simulink model "IEEE9_case"  (R2024b)
settings: Solver=FixedStepAuto  StartTime=0  StopTime=5  FixedStep=1e-7  RelTol=1e-3
values from neighbouring files (symbols this model uses):
  SG_D_1_D = 0.01056    [IEEE9_case_parameters.m]    (also in case1_parameters.m; case2_parameters.m; case3_parameters.m; case4_parameters.m)
  SG_D_1_EnableSaturation = 0    [IEEE9_case_parameters.m]    (also in case1_parameters.m; case2_parameters.m; case3_parameters.m; case4_parameters.m)
  SG_D_1_f0 = 60    [IEEE9_case_parameters.m]    (also in case1_parameters.m; case2_parameters.m; case3_parameters.m; case4_parameters.m)
  SG_D_1_H = 7.5    [IEEE9_case_parameters.m]    (also in case1_parameters.m; case2_parameters.m; case3_parameters.m; case4_parameters.m)
  SG_D_1_K_A = 20    [IEEE9_case_parameters.m]    (also in case1_parameters.m; case2_parameters.m; case3_parameters.m; case4_parameters.m)
  SG_D_1_K_E = 1.000000e+1    (= 10)    [IEEE9_case_parameters.m]    (also in case1_parameters.m; case2_parameters.m; case3_parameters.m; case4_parameters.m)
  SG_D_1_K_F = 2.363    [IEEE9_case_parameters.m]    (also in case1_parameters.m; case2_parameters.m; case3_parameters.m; case4_parameters.m)
  SG_D_1_K_s = 0.5    [IEEE9_case_parameters.m]    (also in case1_parameters.m = 5; case2_parameters.m = 5; case3_parameters.m = 5; case4_parameters.m = 5)
  SG_D_1_R_a = 0.001088    [IEEE9_case_parameters.m]    (also in case1_parameters.m; case2_parameters.m; case3_parameters.m; case4_parameters.m)
  SG_D_1_S_A = 1    [IEEE9_case_parameters.m]    (also in case1_parameters.m; case2_parameters.m; case3_parameters.m; case4_parameters.m)
  SG_D_1_S_B = 0.103    [IEEE9_case_parameters.m]    (also in case1_parameters.m; case2_parameters.m; case3_parameters.m; case4_parameters.m)
  SG_D_1_S_N = 10.659857    [IEEE9_case_parameters.m]    (also in case1_parameters.m; case2_parameters.m; case3_parameters.m; case4_parameters.m)
  SG_D_1_SpeedPara = 200    [IEEE9_case_parameters.m]    (also in case1_parameters.m; case2_parameters.m; case3_parameters.m; case4_parameters.m)
  SG_D_1_T_0 = 0.720173    [IEEE9_case_parameters.m]    (also in case1_parameters.m = 0.755522; case2_parameters.m = 0.808931; case3_parameters.m = 0.869402; case4_parameters.m = 0.729316)
  SG_D_1_T_1 = 0.3    [IEEE9_case_parameters.m]    (also in case1_parameters.m; case2_parameters.m; case3_parameters.m; case4_parameters.m)
  SG_D_1_T_2 = 0.05    [IEEE9_case_parameters.m]    (also in case1_parameters.m; case2_parameters.m; case3_parameters.m; case4_parameters.m)
  SG_D_1_T_3 = 0.02    [IEEE9_case_parameters.m]    (also in case1_parameters.m; case2_parameters.m; case3_parameters.m; case4_parameters.m)
  SG_D_1_T_4 = 0.005    [IEEE9_case_parameters.m]    (also in case1_parameters.m; case2_parameters.m; case3_parameters.m; case4_parameters.m)
  SG_D_1_T_A = 0.02    [IEEE9_case_parameters.m]    (also in case1_parameters.m; case2_parameters.m; case3_parameters.m; case4_parameters.m)
  SG_D_1_T_dd = 8.000000e+0    (= 8)    [IEEE9_case_parameters.m]    (also in case1_parameters.m; case2_parameters.m; case3_parameters.m; case4_parameters.m)
  SG_D_1_T_ddd = 0.04    [IEEE9_case_parameters.m]    (also in case1_parameters.m; case2_parameters.m; case3_parameters.m; case4_parameters.m)
  SG_D_1_T_E = 0.314    [IEEE9_case_parameters.m]    (also in case1_parameters.m; case2_parameters.m; case3_parameters.m; case4_parameters.m)
  SG_D_1_T_F = 0.35    [IEEE9_case_parameters.m]    (also in case1_parameters.m; case2_parameters.m; case3_parameters.m; case4_parameters.m)
  SG_D_1_T_qd = 0.8    [IEEE9_case_parameters.m]    (also in case1_parameters.m; case2_parameters.m; case3_parameters.m; case4_parameters.m)
  SG_D_1_T_qdd = 0.02    [IEEE9_case_parameters.m]    (also in case1_parameters.m; case2_parameters.m; case3_parameters.m; case4_parameters.m)
  SG_D_1_T_speed = 0.1    [IEEE9_case_parameters.m]    (also in case1_parameters.m = 200; case2_parameters.m = 200; case3_parameters.m = 200; case4_parameters.m = 200)
  SG_D_1_T_w = 0.5    [IEEE9_case_parameters.m]    (also in case1_parameters.m; case2_parameters.m; case3_parameters.m; case4_parameters.m)
  SG_D_1_V_ref = 1.990276    [IEEE9_case_parameters.m]    (also in case1_parameters.m = 2.042296; case2_parameters.m = 2.051388; case3_parameters.m = 2.089584; case4_parameters.m = 2.01845)
  SG_D_1_w_ref = 376.991118    [IEEE9_case_parameters.m]    (also in case1_parameters.m; case2_parameters.m; case3_parameters.m; case4_parameters.m)
  SG_D_1_wb = 6.000000e+1    (= 60)    [IEEE9_case_parameters.m]    (also in case1_parameters.m; case2_parameters.m; case3_parameters.m; case4_parameters.m)
  SG_D_1_x_d = 1.9    [IEEE9_case_parameters.m]    (also in case1_parameters.m; case2_parameters.m; case3_parameters.m; case4_parameters.m)
  SG_D_1_x_dd = 0.302    [IEEE9_case_parameters.m]    (also in case1_parameters.m; case2_parameters.m; case3_parameters.m; case4_parameters.m)
  SG_D_1_x_ddd = 0.204    [IEEE9_case_parameters.m]    (also in case1_parameters.m; case2_parameters.m; case3_parameters.m; case4_parameters.m)
  SG_D_1_x_l = 0.05    [IEEE9_case_parameters.m]    (also in case1_parameters.m; case2_parameters.m; case3_parameters.m; case4_parameters.m)
  SG_D_1_x_q = 1.3    [IEEE9_case_parameters.m]    (also in case1_parameters.m; case2_parameters.m; case3_parameters.m; case4_parameters.m)
  SG_D_1_x_qd = 0.5    [IEEE9_case_parameters.m]    (also in case1_parameters.m; case2_parameters.m; case3_parameters.m; case4_parameters.m)
  SG_D_1_x_qdd = 0.3    [IEEE9_case_parameters.m]    (also in case1_parameters.m; case2_parameters.m; case3_parameters.m; case4_parameters.m)
  SG_D_2_D = 0.02    [IEEE9_case_parameters.m]    (also in case1_parameters.m; case2_parameters.m; case3_parameters.m; case4_parameters.m)
  SG_D_2_EnableSaturation = 0    [IEEE9_case_parameters.m]    (also in case1_parameters.m; case2_parameters.m; case3_parameters.m; case4_parameters.m)
  SG_D_2_f0 = 60    [IEEE9_case_parameters.m]    (also in case1_parameters.m; case2_parameters.m; case3_parameters.m; case4_parameters.m)
  SG_D_2_H = 8.000000e+0    (= 8)    [IEEE9_case_parameters.m]    (also in case1_parameters.m; case2_parameters.m; case3_parameters.m; case4_parameters.m)
  SG_D_2_K_A = 20    [IEEE9_case_parameters.m]    (also in case1_parameters.m; case2_parameters.m; case3_parameters.m; case4_parameters.m)
  SG_D_2_K_E = 1.000000e+1    (= 10)    [IEEE9_case_parameters.m]    (also in case1_parameters.m; case2_parameters.m; case3_parameters.m; case4_parameters.m)
  SG_D_2_K_F = 2.363    [IEEE9_case_parameters.m]    (also in case1_parameters.m; case2_parameters.m; case3_parameters.m; case4_parameters.m)
  SG_D_2_K_s = 0.5    [IEEE9_case_parameters.m]    (also in case1_parameters.m = 4; case2_parameters.m = 4; case3_parameters.m = 4; case4_parameters.m = 4)
  SG_D_2_R_a = 0.001088    [IEEE9_case_parameters.m]    (also in case1_parameters.m; case2_parameters.m; case3_parameters.m; case4_parameters.m)
  SG_D_2_S_A = 1    [IEEE9_case_parameters.m]    (also in case1_parameters.m; case2_parameters.m; case3_parameters.m; case4_parameters.m)
  SG_D_2_S_B = 0.103    [IEEE9_case_parameters.m]    (also in case1_parameters.m; case2_parameters.m; case3_parameters.m; case4_parameters.m)
  SG_D_2_S_N = 10.659857    [IEEE9_case_parameters.m]    (also in case1_parameters.m; case2_parameters.m; case3_parameters.m; case4_parameters.m)
  SG_D_2_SpeedPara = 200    [IEEE9_case_parameters.m]    (also in case1_parameters.m; case2_parameters.m; case3_parameters.m; case4_parameters.m)
  SG_D_2_T_0 = 1.632913    [IEEE9_case_parameters.m]    (also in case1_parameters.m = 1.632925; case2_parameters.m = 1.632915; case3_parameters.m = 1.632914; case4_parameters.m = 1.632927)
  SG_D_2_T_1 = 0.2    [IEEE9_case_parameters.m]    (also in case1_parameters.m; case2_parameters.m; case3_parameters.m; case4_parameters.m)
  SG_D_2_T_2 = 0.05    [IEEE9_case_parameters.m]    (also in case1_parameters.m; case2_parameters.m; case3_parameters.m; case4_parameters.m)
  SG_D_2_T_3 = 0.02    [IEEE9_case_parameters.m]    (also in case1_parameters.m; case2_parameters.m; case3_parameters.m; case4_parameters.m)
  SG_D_2_T_4 = 0.005    [IEEE9_case_parameters.m]    (also in case1_parameters.m; case2_parameters.m; case3_parameters.m; case4_parameters.m)
  SG_D_2_T_A = 0.02    [IEEE9_case_parameters.m]    (also in case1_parameters.m; case2_parameters.m; case3_parameters.m; case4_parameters.m)
  SG_D_2_T_dd = 7.9    [IEEE9_case_parameters.m]    (also in case1_parameters.m; case2_parameters.m; case3_parameters.m; case4_parameters.m)
  SG_D_2_T_ddd = 0.04    [IEEE9_case_parameters.m]    (also in case1_parameters.m; case2_parameters.m; case3_parameters.m; case4_parameters.m)
  SG_D_2_T_E = 0.314    [IEEE9_case_parameters.m]    (also in case1_parameters.m; case2_parameters.m; case3_parameters.m; case4_parameters.m)
  SG_D_2_T_F = 0.35    [IEEE9_case_parameters.m]    (also in case1_parameters.m; case2_parameters.m; case3_parameters.m; case4_parameters.m)
  SG_D_2_T_qd = 0.8    [IEEE9_case_parameters.m]    (also in case1_parameters.m; case2_parameters.m; case3_parameters.m; case4_parameters.m)
  SG_D_2_T_qdd = 0.015    [IEEE9_case_parameters.m]    (also in case1_parameters.m; case2_parameters.m; case3_parameters.m; case4_parameters.m)
  SG_D_2_T_speed = 0.1    [IEEE9_case_parameters.m]    (also in case1_parameters.m = 150; case2_parameters.m = 150; case3_parameters.m = 150; case4_parameters.m = 150)
  SG_D_2_T_w = 0.35    [IEEE9_case_parameters.m]    (also in case1_parameters.m; case2_parameters.m; case3_parameters.m; case4_parameters.m)
  SG_D_2_V_ref = 2.58547    [IEEE9_case_parameters.m]    (also in case1_parameters.m = 2.597896; case2_parameters.m = 2.587136; case3_parameters.m = 2.586042; case4_parameters.m = 2.599679)
  SG_D_2_w_ref = 376.991118    [IEEE9_case_parameters.m]    (also in case1_parameters.m; case2_parameters.m; case3_parameters.m; case4_parameters.m)
  SG_D_2_wb = 6.000000e+1    (= 60)    [IEEE9_case_parameters.m]    (also in case1_parameters.m; case2_parameters.m; case3_parameters.m; case4_parameters.m)
  SG_D_2_x_d = 1.8    [IEEE9_case_parameters.m]    (also in case1_parameters.m; case2_parameters.m; case3_parameters.m; case4_parameters.m)
  SG_D_2_x_dd = 0.302    [IEEE9_case_parameters.m]    (also in case1_parameters.m; case2_parameters.m; case3_parameters.m; case4_parameters.m)
  SG_D_2_x_ddd = 0.204    [IEEE9_case_parameters.m]    (also in case1_parameters.m; case2_parameters.m; case3_parameters.m; case4_parameters.m)
  SG_D_2_x_l = 0.05    [IEEE9_case_parameters.m]    (also in case1_parameters.m; case2_parameters.m; case3_parameters.m; case4_parameters.m)
  SG_D_2_x_q = 1.25    [IEEE9_case_parameters.m]    (also in case1_parameters.m; case2_parameters.m; case3_parameters.m; case4_parameters.m)
  SG_D_2_x_qd = 0.5    [IEEE9_case_parameters.m]    (also in case1_parameters.m; case2_parameters.m; case3_parameters.m; case4_parameters.m)
  SG_D_2_x_qdd = 0.3    [IEEE9_case_parameters.m]    (also in case1_parameters.m; case2_parameters.m; case3_parameters.m; case4_parameters.m)
  SG_D_3_D = 0.02    [IEEE9_case_parameters.m]    (also in case1_parameters.m; case2_parameters.m; case3_parameters.m; case4_parameters.m)
  SG_D_3_EnableSaturation = 0    [IEEE9_case_parameters.m]    (also in case1_parameters.m; case2_parameters.m; case3_parameters.m; case4_parameters.m)
  SG_D_3_f0 = 60    [IEEE9_case_parameters.m]    (also in case1_parameters.m; case2_parameters.m; case3_parameters.m; case4_parameters.m)
  SG_D_3_H = 7.7    [IEEE9_case_parameters.m]    (also in case1_parameters.m; case2_parameters.m; case3_parameters.m; case4_parameters.m)
  SG_D_3_K_A = 20    [IEEE9_case_parameters.m]    (also in case1_parameters.m; case2_parameters.m; case3_parameters.m; case4_parameters.m)
  SG_D_3_K_E = 1.000000e+1    (= 10)    [IEEE9_case_parameters.m]    (also in case1_parameters.m; case2_parameters.m; case3_parameters.m; case4_parameters.m)
  SG_D_3_K_F = 2.363    [IEEE9_case_parameters.m]    (also in case1_parameters.m; case2_parameters.m; case3_parameters.m; case4_parameters.m)
  SG_D_3_K_s = 0.2    [IEEE9_case_parameters.m]    (also in case1_parameters.m = 2; case2_parameters.m = 2; case3_parameters.m = 2; case4_parameters.m = 2)
  SG_D_3_R_a = 0.001088    [IEEE9_case_parameters.m]    (also in case1_parameters.m; case2_parameters.m; case3_parameters.m; case4_parameters.m)
  SG_D_3_S_A = 1    [IEEE9_case_parameters.m]    (also in case1_parameters.m; case2_parameters.m; case3_parameters.m; case4_parameters.m)
  SG_D_3_S_B = 0.103    [IEEE9_case_parameters.m]    (also in case1_parameters.m; case2_parameters.m; case3_parameters.m; case4_parameters.m)
  SG_D_3_S_N = 10.659857    [IEEE9_case_parameters.m]    (also in case1_parameters.m; case2_parameters.m; case3_parameters.m; case4_parameters.m)
  SG_D_3_SpeedPara = 200    [IEEE9_case_parameters.m]    (also in case1_parameters.m; case2_parameters.m; case3_parameters.m; case4_parameters.m)
  SG_D_3_T_0 = 0.850788    [IEEE9_case_parameters.m]    (also in case1_parameters.m = 0.850786; case2_parameters.m = 0.850787; case3_parameters.m; case4_parameters.m = 0.850786)
  SG_D_3_T_1 = 0.2    [IEEE9_case_parameters.m]    (also in case1_parameters.m; case2_parameters.m; case3_parameters.m; case4_parameters.m)
  SG_D_3_T_2 = 0.05    [IEEE9_case_parameters.m]    (also in case1_parameters.m; case2_parameters.m; case3_parameters.m; case4_parameters.m)
  SG_D_3_T_3 = 0.02    [IEEE9_case_parameters.m]    (also in case1_parameters.m; case2_parameters.m; case3_parameters.m; case4_parameters.m)
  SG_D_3_T_4 = 0.005    [IEEE9_case_parameters.m]    (also in case1_parameters.m; case2_parameters.m; case3_parameters.m; case4_parameters.m)
  SG_D_3_T_A = 0.02    [IEEE9_case_parameters.m]    (also in case1_parameters.m; case2_parameters.m; case3_parameters.m; case4_parameters.m)
  SG_D_3_T_dd = 8.1    [IEEE9_case_parameters.m]    (also in case1_parameters.m; case2_parameters.m; case3_parameters.m; case4_parameters.m)
  SG_D_3_T_ddd = 0.04    [IEEE9_case_parameters.m]    (also in case1_parameters.m; case2_parameters.m; case3_parameters.m; case4_parameters.m)
  SG_D_3_T_E = 0.314    [IEEE9_case_parameters.m]    (also in case1_parameters.m; case2_parameters.m; case3_parameters.m; case4_parameters.m)
  SG_D_3_T_F = 0.35    [IEEE9_case_parameters.m]    (also in case1_parameters.m; case2_parameters.m; case3_parameters.m; case4_parameters.m)
  SG_D_3_T_qd = 0.8    [IEEE9_case_parameters.m]    (also in case1_parameters.m; case2_parameters.m; case3_parameters.m; case4_parameters.m)
  SG_D_3_T_qdd = 0.015    [IEEE9_case_parameters.m]    (also in case1_parameters.m; case2_parameters.m; case3_parameters.m; case4_parameters.m)
  SG_D_3_T_speed = 0.1    [IEEE9_case_parameters.m]    (also in case1_parameters.m = 180; case2_parameters.m = 180; case3_parameters.m = 180; case4_parameters.m = 180)
  SG_D_3_T_w = 0.4    [IEEE9_case_parameters.m]    (also in case1_parameters.m; case2_parameters.m; case3_parameters.m; case4_parameters.m)
  SG_D_3_V_ref = 1.892727    [IEEE9_case_parameters.m]    (also in case1_parameters.m = 1.906439; case2_parameters.m = 1.895535; case3_parameters.m = 1.892105; case4_parameters.m = 1.906598)
  SG_D_3_w_ref = 376.991118    [IEEE9_case_parameters.m]    (also in case1_parameters.m; case2_parameters.m; case3_parameters.m; case4_parameters.m)
  SG_D_3_wb = 6.000000e+1    (= 60)    [IEEE9_case_parameters.m]    (also in case1_parameters.m; case2_parameters.m; case3_parameters.m; case4_parameters.m)
  SG_D_3_x_d = 1.85    [IEEE9_case_parameters.m]    (also in case1_parameters.m; case2_parameters.m; case3_parameters.m; case4_parameters.m)
  SG_D_3_x_dd = 0.302    [IEEE9_case_parameters.m]    (also in case1_parameters.m; case2_parameters.m; case3_parameters.m; case4_parameters.m)
  SG_D_3_x_ddd = 0.204    [IEEE9_case_parameters.m]    (also in case1_parameters.m; case2_parameters.m; case3_parameters.m; case4_parameters.m)
  SG_D_3_x_l = 0.05    [IEEE9_case_parameters.m]    (also in case1_parameters.m; case2_parameters.m; case3_parameters.m; case4_parameters.m)
  SG_D_3_x_q = 1.2    [IEEE9_case_parameters.m]    (also in case1_parameters.m; case2_parameters.m; case3_parameters.m; case4_parameters.m)
  SG_D_3_x_qd = 0.5    [IEEE9_case_parameters.m]    (also in case1_parameters.m; case2_parameters.m; case3_parameters.m; case4_parameters.m)
  SG_D_3_x_qdd = 0.3    [IEEE9_case_parameters.m]    (also in case1_parameters.m; case2_parameters.m; case3_parameters.m; case4_parameters.m)
(part 11 of 12)

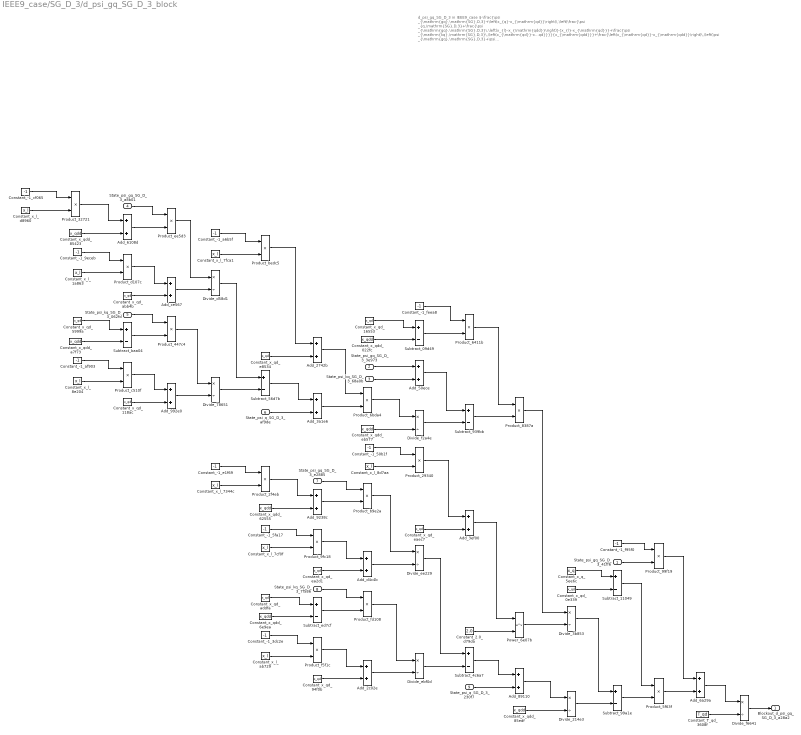
== system IEEE9_case/SG_D_3/d_psi_gq_SG_D_3_block ==
  note: d_psi_gq_SG_D_3 in IEEE9_case
      | $-\frac{\psi _{\mathrm{gq},\mathrm{SG},D,3}+\left(x_{q}-x_{\mathrm{qd}}\right)\,\left(\frac{\psi _{q,\mathrm{SG},D,3}+\frac{\psi _{\mathrm{gq},\mathrm{SG},D,3}\,\left(x_{l}-x_{\mathrm{qdd}}\right)}{x_{l}-x_{\mathrm{qd}}}+\frac{\psi _{\mathrm{kq},\mathrm{SG},D,3}\,\left(x_{\mathrm{qd}}-x_{\mathrm{qdd}}\right)}{x_{l}-x_{\mathrm{qd}}}}{x_{\mathrm{qdd}}}+\frac{\left(x_{\mathrm{qd}}-x_{\mathrm{qdd}}\right)\,\left(\psi _{\mathrm{gq},\mathrm{SG},D,3}+\psi _{\mathrm{kq},\mathrm{SG},D,3}+\frac{\left(x_{l}-x_{\mathrm{qd}}\right)\,\left(\psi _{q,\mathrm{SG},D,3}+\frac{\psi _{\mathrm{gq},\mathrm{SG},D,3}\,\left(x_{l}-x_{\mathrm{qdd}}\right)}{x_{l}-x_{\mathrm{qd}}}+\frac{\psi _{\mathrm{kq},\mathrm{SG},D,3}\,\left(x_{\mathrm{qd}}-x_{\mathrm{qdd}}\right)}{x_{l}-x_{\mathrm{qd}}}\right)}{x_{\mathrm{qdd}}}\right)}{{\left(x_{l}-x_{\mathrm{qd}}\right)}^2}\right)}{T_{\mathrm{qd}}}$
      | Automatically generated on 2025-11-01 08:49:54 .
  State_psi_gq_SG_D_3_41ff6 : Inport
  State_psi_gq_SG_D_3_3e973 : Inport  Port=2
  State_psi_kq_SG_D_3_68a0b : Inport  Port=3
  State_psi_gq_SG_D_3_a8b01 : Inport  Port=4
  State_psi_kq_SG_D_3_062fd : Inport  Port=5
  State_psi_q_SG_D_3_af9de : Inport  Port=6
  State_psi_gq_SG_D_3_e2885 : Inport  Port=7
  State_psi_kq_SG_D_3_7f586 : Inport  Port=8
  State_psi_q_SG_D_3_230f7 : Inport  Port=9
  Add_2742b : Sum
  Add_2c02e : Sum
  Add_3a1e6 : Sum
  Add_3ef00 : Sum
  Add_50ece : Sum
  Add_6108d : Sum
  Add_6a29a : Sum
  Add_89110 : Sum
  Add_9238c : Sum
  Add_992e0 : Sum
  Add_ce567 : Sum
  Add_d4c4b : Sum
  Constant_-1_3dc2e : Constant  Value=-1
  Constant_-1_50b1f : Constant  Value=-1
  Constant_-1_5fa17 : Constant  Value=-1
  Constant_-1_9eceb : Constant  Value=-1
  Constant_-1_a6b5f : Constant  Value=-1
  Constant_-1_af903 : Constant  Value=-1
  Constant_-1_cf065 : Constant  Value=-1
  Constant_-1_e1f69 : Constant  Value=-1
  Constant_-1_f95f0 : Constant  Value=-1
  Constant_-1_feea8 : Constant  Value=-1
  Constant_2.0_d79da : Constant  Value=2.0
  Constant_T_qd_3608f : Constant  Value=T_qd
  Constant_x_l_1a863 : Constant  Value=x_l
  Constant_x_l_7344c : Constant  Value=x_l
  Constant_x_l_7cf0f : Constant  Value=x_l
  Constant_x_l_7fca1 : Constant  Value=x_l
  Constant_x_l_8d7aa : Constant  Value=x_l
  Constant_x_l_8e204 : Constant  Value=x_l
  Constant_x_l_ab729 : Constant  Value=x_l
  Constant_x_l_d8960 : Constant  Value=x_l
  Constant_x_q_5ee6c : Constant  Value=x_q
  Constant_x_qd_0e339 : Constant  Value=x_qd
  Constant_x_qd_118ac : Constant  Value=x_qd
  Constant_x_qd_16553 : Constant  Value=x_qd
  Constant_x_qd_5999a : Constant  Value=x_qd
  Constant_x_qd_94f0b : Constant  Value=x_qd
  Constant_x_qd_abb4b : Constant  Value=x_qd
  Constant_x_qd_addfa : Constant  Value=x_qd
  Constant_x_qd_e8534 : Constant  Value=x_qd
  Constant_x_qd_ea2d1 : Constant  Value=x_qd
  Constant_x_qd_eaec7 : Constant  Value=x_qd
  Constant_x_qdd_022fc : Constant  Value=x_qdd
  Constant_x_qdd_62555 : Constant  Value=x_qdd
  Constant_x_qdd_6e9ea : Constant  Value=x_qdd
  Constant_x_qdd_85423 : Constant  Value=x_qdd
  Constant_x_qdd_85edf : Constant  Value=x_qdd
  Constant_x_qdd_a7f73 : Constant  Value=x_qdd
  Constant_x_qdd_eb577 : Constant  Value=x_qdd
  Divide_214e3 : Product  Inputs=*/
  Divide_3b853 : Product  Inputs=*/
  Divide_78651 : Product  Inputs=*/
  Divide_d58d1 : Product  Inputs=*/
  Divide_ebf0d : Product  Inputs=*/
  Divide_ee229 : Product  Inputs=*/
  Divide_f2a4e : Product  Inputs=*/
  Divide_f6641 : Product  Inputs=*/
  Power_6e07b : Math  Operator=pow
  Product_29340 : Product
  Product_2f4eb : Product
  Product_32721 : Product
  Product_447c4 : Product
  Product_5f63f : Product
  Product_6411b : Product
  Product_6bda4 : Product
  Product_8387a : Product
  Product_99f19 : Product
  Product_9fc18 : Product
  Product_b9e2a : Product
  Product_bedc5 : Product
  Product_c510f : Product
  Product_d107c : Product
  Product_ee5d3 : Product
  Product_f5f1c : Product
  Product_fd108 : Product
  Subtract_09d49 : Sum  Inputs=+-
  Subtract_11049 : Sum  Inputs=+-
  Subtract_4c6a7 : Sum  Inputs=+-
  Subtract_56d7b : Sum  Inputs=+-
  Subtract_939bb : Sum  Inputs=+-
  Subtract_99a1e : Sum  Inputs=+-
  Subtract_baa04 : Sum  Inputs=+-
  Subtract_ed7cf : Sum  Inputs=+-
  Blockout_d_psi_gq_SG_D_3_a28a2 : Outport
  wires:
  Constant_x_l_8d7aa/1 -> Product_29340/2
  Constant_x_qd_5999a/1 -> Subtract_baa04/1
  Add_2742b/1 -> Product_6bda4/1
  Constant_-1_cf065/1 -> Product_32721/1
  Add_6108d/1 -> Product_ee5d3/2
  Constant_x_qdd_a7f73/1 -> Subtract_baa04/2
  Constant_x_qd_e8534/1 -> Add_2742b/2
  Constant_x_l_d8960/1 -> Product_32721/2
  Constant_x_l_1a863/1 -> Product_d107c/2
  Add_2c02e/1 -> Divide_ebf0d/2
  State_psi_kq_SG_D_3_68a0b/1 -> Add_50ece/2
  Constant_x_qdd_85423/1 -> Add_6108d/2
  Product_32721/1 -> Add_6108d/1
  Constant_x_qd_94f0b/1 -> Add_2c02e/2
  Product_6411b/1 -> Product_8387a/1
  Constant_-1_e1f69/1 -> Product_2f4eb/1
  Constant_-1_9eceb/1 -> Product_d107c/1
  Constant_-1_af903/1 -> Product_c510f/1
  Constant_x_l_8e204/1 -> Product_c510f/2
  Constant_-1_feea8/1 -> Product_6411b/1
  Constant_-1_f95f0/1 -> Product_99f19/1
  State_psi_gq_SG_D_3_a8b01/1 -> Product_ee5d3/1
  Product_2f4eb/1 -> Add_9238c/1
  Product_d107c/1 -> Add_ce567/1
  Product_f5f1c/1 -> Add_2c02e/1
  Constant_x_qd_abb4b/1 -> Add_ce567/2
  Constant_-1_5fa17/1 -> Product_9fc18/1
  State_psi_kq_SG_D_3_062fd/1 -> Product_447c4/1
  Subtract_baa04/1 -> Product_447c4/2
  Product_c510f/1 -> Add_992e0/1
  Add_9238c/1 -> Product_b9e2a/2
  Add_ce567/1 -> Divide_d58d1/2
  Constant_x_qd_118ac/1 -> Add_992e0/2
  Product_ee5d3/1 -> Divide_d58d1/1
  Constant_T_qd_3608f/1 -> Divide_f6641/2
  Product_9fc18/1 -> Add_d4c4b/1
  Product_447c4/1 -> Divide_78651/1
  Product_fd108/1 -> Divide_ebf0d/1
  Add_992e0/1 -> Divide_78651/2
  Constant_-1_a6b5f/1 -> Product_bedc5/1
  Constant_x_qdd_eb577/1 -> Divide_f2a4e/2
  Constant_x_l_7fca1/1 -> Product_bedc5/2
  Divide_d58d1/1 -> Subtract_56d7b/1
  Constant_x_qd_0e339/1 -> Subtract_11049/2
  Add_d4c4b/1 -> Divide_ee229/2
  Divide_78651/1 -> Subtract_56d7b/2
  Constant_x_l_7344c/1 -> Product_2f4eb/2
  Product_bedc5/1 -> Add_2742b/1
  Constant_-1_50b1f/1 -> Product_29340/1
  Constant_x_l_7cf0f/1 -> Product_9fc18/2
  Subtract_56d7b/1 -> Add_3a1e6/1
  State_psi_q_SG_D_3_af9de/1 -> Add_3a1e6/2
  Constant_-1_3dc2e/1 -> Product_f5f1c/1
  Constant_x_qdd_62555/1 -> Add_9238c/2
  Constant_x_qd_addfa/1 -> Subtract_ed7cf/1
  Constant_x_qdd_6e9ea/1 -> Subtract_ed7cf/2
  Constant_x_l_ab729/1 -> Product_f5f1c/2
  Add_3a1e6/1 -> Product_6bda4/2
  Constant_x_qdd_022fc/1 -> Subtract_09d49/2
  State_psi_gq_SG_D_3_e2885/1 -> Product_b9e2a/1
  Constant_x_qd_ea2d1/1 -> Add_d4c4b/2
  Divide_3b853/1 -> Subtract_99a1e/1
  State_psi_kq_SG_D_3_7f586/1 -> Product_fd108/1
  Subtract_ed7cf/1 -> Product_fd108/2
  Constant_x_qd_16553/1 -> Subtract_09d49/1
  State_psi_gq_SG_D_3_3e973/1 -> Add_50ece/1
  Product_6bda4/1 -> Divide_f2a4e/1
  Product_b9e2a/1 -> Divide_ee229/1
  Subtract_09d49/1 -> Product_6411b/2
  Add_50ece/1 -> Subtract_939bb/1
  Divide_f2a4e/1 -> Subtract_939bb/2
  Product_29340/1 -> Add_3ef00/1
  Constant_x_qd_eaec7/1 -> Add_3ef00/2
  Divide_ee229/1 -> Subtract_4c6a7/1
  Divide_ebf0d/1 -> Subtract_4c6a7/2
  Subtract_939bb/1 -> Product_8387a/2
  Add_3ef00/1 -> Power_6e07b/1
  Constant_2.0_d79da/1 -> Power_6e07b/2
  Subtract_4c6a7/1 -> Add_89110/1
  State_psi_q_SG_D_3_230f7/1 -> Add_89110/2
  Product_8387a/1 -> Divide_3b853/1
  Power_6e07b/1 -> Divide_3b853/2
  Add_89110/1 -> Divide_214e3/1
  Constant_x_qdd_85edf/1 -> Divide_214e3/2
  Constant_x_q_5ee6c/1 -> Subtract_11049/1
  Divide_214e3/1 -> Subtract_99a1e/2
  State_psi_gq_SG_D_3_41ff6/1 -> Product_99f19/2
  Subtract_11049/1 -> Product_5f63f/1
  Subtract_99a1e/1 -> Product_5f63f/2
  Product_99f19/1 -> Add_6a29a/1
  Product_5f63f/1 -> Add_6a29a/2
  Add_6a29a/1 -> Divide_f6641/1
  Divide_f6641/1 -> Blockout_d_psi_gq_SG_D_3_a28a2/1

== system IEEE9_case/SG_D_3/d_psi_kq_SG_D_3_block ==
  note: d_psi_kq_SG_D_3 in IEEE9_case
      | $-\frac{\psi _{\mathrm{gq},\mathrm{SG},D,3}+\psi _{\mathrm{kq},\mathrm{SG},D,3}+\frac{\left(x_{l}-x_{\mathrm{qd}}\right)\,\left(\psi _{q,\mathrm{SG},D,3}+\frac{\psi _{\mathrm{gq},\mathrm{SG},D,3}\,\left(x_{l}-x_{\mathrm{qdd}}\right)}{x_{l}-x_{\mathrm{qd}}}+\frac{\psi _{\mathrm{kq},\mathrm{SG},D,3}\,\left(x_{\mathrm{qd}}-x_{\mathrm{qdd}}\right)}{x_{l}-x_{\mathrm{qd}}}\right)}{x_{\mathrm{qdd}}}}{T_{\mathrm{qdd}}}$
      | Automatically generated on 2025-11-01 08:49:56 .
  State_psi_gq_SG_D_3_86c60 : Inport
  State_psi_kq_SG_D_3_0238a : Inport  Port=2
  State_psi_gq_SG_D_3_7b374 : Inport  Port=3
  State_psi_kq_SG_D_3_310cd : Inport  Port=4
  State_psi_q_SG_D_3_2e3f0 : Inport  Port=5
  Add_0f51c : Sum
  Add_16649 : Sum
  Add_7bf3d : Sum
  Add_affbb : Sum
  Add_c9ad0 : Sum
  Add_dd819 : Sum
  Constant_-1_28cd3 : Constant  Value=-1
  Constant_-1_79d5f : Constant  Value=-1
  Constant_-1_bc8bb : Constant  Value=-1
  Constant_-1_c8bdb : Constant  Value=-1
  Constant_-1_f2606 : Constant  Value=-1
  Constant_T_qdd_0e0b0 : Constant  Value=T_qdd
  Constant_x_l_08161 : Constant  Value=x_l
  Constant_x_l_7f51f : Constant  Value=x_l
  Constant_x_l_b2bba : Constant  Value=x_l
  Constant_x_l_d9a1b : Constant  Value=x_l
  Constant_x_qd_11e02 : Constant  Value=x_qd
  Constant_x_qd_2de2d : Constant  Value=x_qd
  Constant_x_qd_4e3c6 : Constant  Value=x_qd
  Constant_x_qd_7fcd4 : Constant  Value=x_qd
  Constant_x_qdd_612fe : Constant  Value=x_qdd
  Constant_x_qdd_7e914 : Constant  Value=x_qdd
  Constant_x_qdd_af8a6 : Constant  Value=x_qdd
  Divide_26b67 : Product  Inputs=*/
  Divide_30de3 : Product  Inputs=*/
  Divide_57d74 : Product  Inputs=*/
  Divide_ae6c8 : Product  Inputs=*/
  Product_2d578 : Product
  Product_363c3 : Product
  Product_38e12 : Product
  Product_3aff0 : Product
  Product_7f603 : Product
  Product_8ac75 : Product
  Product_bb545 : Product
  Product_f921b : Product
  Subtract_3cba1 : Sum  Inputs=+-
  Subtract_3d5a0 : Sum  Inputs=+-
  Subtract_534ed : Sum  Inputs=+-
  Blockout_d_psi_kq_SG_D_3_0e0d5 : Outport
  wires:
  State_psi_q_SG_D_3_2e3f0/1 -> Add_16649/2
  Constant_-1_28cd3/1 -> Product_f921b/1
  Constant_-1_f2606/1 -> Product_38e12/1
  Constant_-1_79d5f/1 -> Product_bb545/1
  Constant_x_l_08161/1 -> Product_f921b/2
  Constant_x_qdd_7e914/1 -> Add_dd819/2
  Product_3aff0/1 -> Add_7bf3d/1
  Constant_x_l_7f51f/1 -> Product_38e12/2
  Constant_x_qd_2de2d/1 -> Subtract_3cba1/1
  Product_38e12/1 -> Add_dd819/1
  Constant_x_l_d9a1b/1 -> Product_363c3/2
  Constant_x_qdd_af8a6/1 -> Subtract_3cba1/2
  Constant_-1_bc8bb/1 -> Product_3aff0/1
  Constant_x_l_b2bba/1 -> Product_3aff0/2
  State_psi_gq_SG_D_3_7b374/1 -> Product_7f603/1
  Add_dd819/1 -> Product_7f603/2
  Add_16649/1 -> Product_2d578/2
  Product_f921b/1 -> Add_affbb/1
  Constant_x_qd_7fcd4/1 -> Add_affbb/2
  State_psi_kq_SG_D_3_310cd/1 -> Product_8ac75/1
  Subtract_3cba1/1 -> Product_8ac75/2
  Add_affbb/1 -> Divide_ae6c8/2
  Constant_x_qd_11e02/1 -> Add_7bf3d/2
  Product_7f603/1 -> Divide_ae6c8/1
  Product_8ac75/1 -> Divide_26b67/1
  Add_7bf3d/1 -> Divide_26b67/2
  Constant_-1_c8bdb/1 -> Product_363c3/1
  Divide_ae6c8/1 -> Subtract_534ed/1
  Add_0f51c/1 -> Divide_57d74/1
  Divide_26b67/1 -> Subtract_534ed/2
  Divide_57d74/1 -> Blockout_d_psi_kq_SG_D_3_0e0d5/1
  Product_363c3/1 -> Add_c9ad0/1
  Constant_x_qd_4e3c6/1 -> Add_c9ad0/2
  Subtract_534ed/1 -> Add_16649/1
  State_psi_gq_SG_D_3_86c60/1 -> Product_bb545/2
  Add_c9ad0/1 -> Product_2d578/1
  Constant_T_qdd_0e0b0/1 -> Divide_57d74/2
  Product_bb545/1 -> Subtract_3d5a0/1
  State_psi_kq_SG_D_3_0238a/1 -> Subtract_3d5a0/2
  Product_2d578/1 -> Divide_30de3/1
  Constant_x_qdd_612fe/1 -> Divide_30de3/2
  Subtract_3d5a0/1 -> Add_0f51c/1
  Divide_30de3/1 -> Add_0f51c/2

== system IEEE9_case/SG_D_3/d_psi_q_SG_D_3_block ==
  note: d_psi_q_SG_D_3 in IEEE9_case
      | $2\,\pi \,f_{0}\,\left(v_{d,\mathrm{SG},D,3}\,\cos\left(\theta _{\mathrm{SG},D,3}\right)+v_{q,\mathrm{SG},D,3}\,\sin\left(\theta _{\mathrm{SG},D,3}\right)-\frac{R_{a}\,\left(\psi _{q,\mathrm{SG},D,3}+\frac{\psi _{\mathrm{gq},\mathrm{SG},D,3}\,\left(x_{l}-x_{\mathrm{qdd}}\right)}{x_{l}-x_{\mathrm{qd}}}+\frac{\psi _{\mathrm{kq},\mathrm{SG},D,3}\,\left(x_{\mathrm{qd}}-x_{\mathrm{qdd}}\right)}{x_{l}-x_{\mathrm{qd}}}\right)}{x_{\mathrm{qdd}}}-\frac{\psi _{d,\mathrm{SG},D,3}\,w_{\mathrm{SG},D,3}}{2\,f_{0}\,\pi }\right)$
      | Automatically generated on 2025-11-01 08:49:41 .
  State_psi_gq_SG_D_3_cf09c : Inport
  State_psi_kq_SG_D_3_c8fad : Inport  Port=2
  State_psi_q_SG_D_3_7832e : Inport  Port=3
  Input_v_d_SG_D_3_4ab93 : Inport  Port=4
  State_theta_SG_D_3_c9886 : Inport  Port=5
  Input_v_q_SG_D_3_8644a : Inport  Port=6
  State_theta_SG_D_3_067ed : Inport  Port=7
  State_psi_d_SG_D_3_bc54d : Inport  Port=8
  State_w_SG_D_3_7541e : Inport  Port=9
  Add_08b14 : Sum
  Add_0bbb5 : Sum
  Add_55f62 : Sum
  Add_6e916 : Sum
  Add_bac07 : Sum
  Constant_-1_17af4 : Constant  Value=-1
  Constant_-1_18eb3 : Constant  Value=-1
  Constant_-1_c534c : Constant  Value=-1
  Constant_-2.0_636ca : Constant  Value=-2.0
  Constant_2.0_d3a80 : Constant  Value=2.0
  Constant_R_a_46d95 : Constant  Value=R_a
  Constant_f0_66d84 : Constant  Value=f0
  Constant_f0_85878 : Constant  Value=f0
  Constant_pi_5c30a : Constant  Value=pi
  Constant_pi_b2111 : Constant  Value=pi
  Constant_x_l_14cb5 : Constant  Value=x_l
  Constant_x_l_77da6 : Constant  Value=x_l
  Constant_x_l_a47c6 : Constant  Value=x_l
  Constant_x_qd_3d3c9 : Constant  Value=x_qd
  Constant_x_qd_44bfa : Constant  Value=x_qd
  Constant_x_qd_851af : Constant  Value=x_qd
  Constant_x_qdd_1dace : Constant  Value=x_qdd
  Constant_x_qdd_6cc31 : Constant  Value=x_qdd
  Constant_x_qdd_6f1ed : Constant  Value=x_qdd
  Divide_21caf : Product  Inputs=*/
  Divide_73856 : Product  Inputs=*/
  Divide_78272 : Product  Inputs=*/
  Divide_b5021 : Product  Inputs=*/
  MathFunc_cos_19683 : Trigonometry  Operator=cos
  MathFunc_sin_0ec18 : Trigonometry
  Product_273de : Product
  Product_3dd0f : Product
  Product_41f43 : Product
  Product_44d74 : Product
  Product_51ca2 : Product
  Product_66925 : Product
  Product_8e5c1 : Product
  Product_92f5f : Product
  Product_93df0 : Product
  Product_b1626 : Product
  Product_c77d2 : Product
  Product_ca7a6 : Product
  Product_d4d8c : Product
  Product_e6fd6 : Product
  Subtract_1b9a6 : Sum  Inputs=+-
  Subtract_421cd : Sum  Inputs=+-
  Subtract_6231f : Sum  Inputs=+-
  Subtract_c1c12 : Sum  Inputs=+-
  Blockout_d_psi_q_SG_D_3_417db : Outport
  wires:
  Constant_x_qd_3d3c9/1 -> Subtract_1b9a6/1
  Constant_pi_b2111/1 -> Product_41f43/2
  Product_92f5f/1 -> Divide_21caf/1
  Constant_x_l_14cb5/1 -> Product_3dd0f/2
  Constant_f0_85878/1 -> Product_ca7a6/2
  State_w_SG_D_3_7541e/1 -> Product_273de/2
  Constant_-1_c534c/1 -> Product_93df0/1
  Constant_x_qdd_6f1ed/1 -> Add_6e916/2
  Input_v_d_SG_D_3_4ab93/1 -> Product_8e5c1/1
  Constant_x_qdd_1dace/1 -> Subtract_1b9a6/2
  Constant_x_l_a47c6/1 -> Product_93df0/2
  Divide_73856/1 -> Add_bac07/2
  Product_93df0/1 -> Add_6e916/1
  Constant_2.0_d3a80/1 -> Product_41f43/1
  Add_08b14/1 -> Product_92f5f/2
  Constant_-1_17af4/1 -> Product_3dd0f/1
  Constant_x_qd_44bfa/1 -> Add_55f62/2
  Constant_-1_18eb3/1 -> Product_44d74/1
  Subtract_6231f/1 -> Subtract_421cd/1
  Constant_x_l_77da6/1 -> Product_44d74/2
  Subtract_421cd/1 -> Add_bac07/1
  Constant_f0_66d84/1 -> Product_d4d8c/2
  State_theta_SG_D_3_067ed/1 -> MathFunc_sin_0ec18/1
  Constant_x_qd_851af/1 -> Add_0bbb5/2
  State_psi_gq_SG_D_3_cf09c/1 -> Product_66925/1
  Add_6e916/1 -> Product_66925/2
  Product_41f43/1 -> Product_d4d8c/1
  Product_3dd0f/1 -> Add_0bbb5/1
  State_psi_kq_SG_D_3_c8fad/1 -> Product_e6fd6/1
  Subtract_1b9a6/1 -> Product_e6fd6/2
  Product_44d74/1 -> Add_55f62/1
  MathFunc_sin_0ec18/1 -> Product_c77d2/2
  Product_66925/1 -> Divide_b5021/1
  Product_d4d8c/1 -> Divide_73856/2
  Add_0bbb5/1 -> Divide_b5021/2
  Product_e6fd6/1 -> Divide_78272/1
  Add_55f62/1 -> Divide_78272/2
  Input_v_q_SG_D_3_8644a/1 -> Product_c77d2/1
  Divide_b5021/1 -> Subtract_c1c12/1
  Subtract_c1c12/1 -> Add_08b14/1
  Divide_78272/1 -> Subtract_c1c12/2
  Divide_21caf/1 -> Subtract_6231f/1
  State_psi_q_SG_D_3_7832e/1 -> Add_08b14/2
  Product_c77d2/1 -> Subtract_421cd/2
  Constant_R_a_46d95/1 -> Product_92f5f/1
  State_theta_SG_D_3_c9886/1 -> MathFunc_cos_19683/1
  Constant_x_qdd_6cc31/1 -> Divide_21caf/2
  MathFunc_cos_19683/1 -> Product_8e5c1/2
  Constant_-2.0_636ca/1 -> Product_b1626/1
  Product_8e5c1/1 -> Subtract_6231f/2
  State_psi_d_SG_D_3_bc54d/1 -> Product_273de/1
  Constant_pi_5c30a/1 -> Product_b1626/2
  Product_273de/1 -> Divide_73856/1
  Product_b1626/1 -> Product_ca7a6/1
  Product_ca7a6/1 -> Product_51ca2/1
  Add_bac07/1 -> Product_51ca2/2
  Product_51ca2/1 -> Blockout_d_psi_q_SG_D_3_417db/1

== system IEEE9_case/SG_D_3/d_theta_SG_D_3_block ==
  note: d_theta_SG_D_3 in IEEE9_case
      | $w_{\mathrm{SG},D,3}-2\,\pi \,f_{0}$
      | Automatically generated on 2025-11-01 08:50:03 .
  State_w_SG_D_3_1039d : Inport
  Add_ed9e2 : Sum
  Constant_-2.0_e92f1 : Constant  Value=-2.0
  Constant_f0_e469c : Constant  Value=f0
  Constant_pi_ec720 : Constant  Value=pi
  Product_abe2d : Product
  Product_acf90 : Product
  Blockout_d_theta_SG_D_3_5365d : Outport
  wires:
  Constant_-2.0_e92f1/1 -> Product_acf90/1
  Constant_pi_ec720/1 -> Product_acf90/2
  State_w_SG_D_3_1039d/1 -> Add_ed9e2/2
  Product_acf90/1 -> Product_abe2d/1
  Constant_f0_e469c/1 -> Product_abe2d/2
  Product_abe2d/1 -> Add_ed9e2/1
  Add_ed9e2/1 -> Blockout_d_theta_SG_D_3_5365d/1

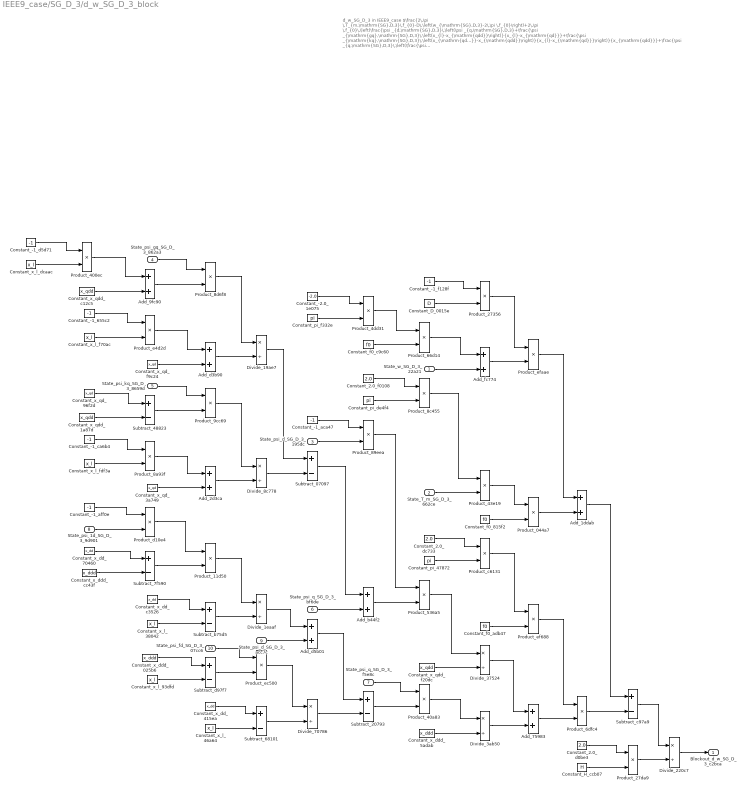
== system IEEE9_case/SG_D_3/d_w_SG_D_3_block ==
  note: d_w_SG_D_3 in IEEE9_case
      | $\frac{2\,\pi \,T_{m,\mathrm{SG},D,3}\,f_{0}-D\,\left(w_{\mathrm{SG},D,3}-2\,\pi \,f_{0}\right)+2\,\pi \,f_{0}\,\left(\frac{\psi _{d,\mathrm{SG},D,3}\,\left(\psi _{q,\mathrm{SG},D,3}+\frac{\psi _{\mathrm{gq},\mathrm{SG},D,3}\,\left(x_{l}-x_{\mathrm{qdd}}\right)}{x_{l}-x_{\mathrm{qd}}}+\frac{\psi _{\mathrm{kq},\mathrm{SG},D,3}\,\left(x_{\mathrm{qd}}-x_{\mathrm{qdd}}\right)}{x_{l}-x_{\mathrm{qd}}}\right)}{x_{\mathrm{qdd}}}+\frac{\psi _{q,\mathrm{SG},D,3}\,\left(\frac{\psi _{\mathrm{1d},\mathrm{SG},D,3}\,\left(x_{\mathrm{dd}}-x_{\mathrm{ddd}}\right)}{x_{\mathrm{dd}}-x_{l}}-\psi _{d,\mathrm{SG},D,3}+\frac{\psi _{\mathrm{fd},\mathrm{SG},D,3}\,\left(x_{\mathrm{ddd}}-x_{l}\right)}{x_{\mathrm{dd}}-x_{l}}\right)}{x_{\mathrm{ddd}}}\right)}{2\,H}$
      | Automatically generated on 2025-11-01 08:50:01 .
  State_w_SG_D_3_22a21 : Inport
  State_T_m_SG_D_3_662ce : Inport  Port=2
  State_psi_d_SG_D_3_195dc : Inport  Port=3
  State_psi_gq_SG_D_3_862a3 : Inport  Port=4
  State_psi_kq_SG_D_3_8659d : Inport  Port=5
  State_psi_q_SG_D_3_bf6de : Inport  Port=6
  State_psi_q_SG_D_3_f5e8c : Inport  Port=7
  State_psi_1d_SG_D_3_9d901 : Inport  Port=8
  State_psi_d_SG_D_3_acc7c : Inport  Port=9
  State_psi_fd_SG_D_3_07cc6 : Inport  Port=10
  Add_1ddab : Sum
  Add_2d3ca : Sum
  Add_75983 : Sum
  Add_9fc90 : Sum
  Add_b44f2 : Sum
  Add_d3b90 : Sum
  Add_d5b01 : Sum
  Add_fc774 : Sum
  Constant_-1_655c2 : Constant  Value=-1
  Constant_-1_aca47 : Constant  Value=-1
  Constant_-1_aff0e : Constant  Value=-1
  Constant_-1_ca6b4 : Constant  Value=-1
  Constant_-1_d5d71 : Constant  Value=-1
  Constant_-1_f128f : Constant  Value=-1
  Constant_-2.0_1e075 : Constant  Value=-2.0
  Constant_2.0_d0be3 : Constant  Value=2.0
  Constant_2.0_dc733 : Constant  Value=2.0
  Constant_2.0_f0108 : Constant  Value=2.0
  Constant_D_0015e : Constant  Value=D
  Constant_H_ccb07 : Constant  Value=H
  Constant_f0_815f2 : Constant  Value=f0
  Constant_f0_adb47 : Constant  Value=f0
  Constant_f0_c9c60 : Constant  Value=f0
  Constant_pi_47872 : Constant  Value=pi
  Constant_pi_de4f4 : Constant  Value=pi
  Constant_pi_f332e : Constant  Value=pi
  Constant_x_dd_415ea : Constant  Value=x_dd
  Constant_x_dd_70460 : Constant  Value=x_dd
  Constant_x_dd_c3526 : Constant  Value=x_dd
  Constant_x_ddd_025b6 : Constant  Value=x_ddd
  Constant_x_ddd_5adab : Constant  Value=x_ddd
  Constant_x_ddd_cc43f : Constant  Value=x_ddd
  Constant_x_l_38042 : Constant  Value=x_l
  Constant_x_l_46a64 : Constant  Value=x_l
  Constant_x_l_93dfd : Constant  Value=x_l
  Constant_x_l_dcaac : Constant  Value=x_l
  Constant_x_l_f70ac : Constant  Value=x_l
  Constant_x_l_fdf3a : Constant  Value=x_l
  Constant_x_qd_3a749 : Constant  Value=x_qd
  Constant_x_qd_96f2d : Constant  Value=x_qd
  Constant_x_qd_f9c24 : Constant  Value=x_qd
  Constant_x_qdd_1a87d : Constant  Value=x_qdd
  Constant_x_qdd_c12c5 : Constant  Value=x_qdd
  Constant_x_qdd_f20dc : Constant  Value=x_qdd
  Divide_19ae7 : Product  Inputs=*/
  Divide_1eaaf : Product  Inputs=*/
  Divide_220c7 : Product  Inputs=*/
  Divide_37524 : Product  Inputs=*/
  Divide_3ab50 : Product  Inputs=*/
  Divide_70786 : Product  Inputs=*/
  Divide_8c778 : Product  Inputs=*/
  Product_044a7 : Product
  Product_11d50 : Product
  Product_27356 : Product
  Product_27da9 : Product
  Product_400ec : Product
  Product_40a83 : Product
  Product_43e19 : Product
  Product_4dd31 : Product
  Product_536a5 : Product
  Product_66d14 : Product
  Product_6dfc4 : Product
  Product_89eea : Product
  Product_8a93f : Product
  Product_8c455 : Product
  Product_8d6f8 : Product
  Product_9cc69 : Product
  Product_c6131 : Product
  Product_d10e4 : Product
  Product_e4d2d : Product
  Product_ec500 : Product
  Product_ef688 : Product
  Product_efaae : Product
  Subtract_07097 : Sum  Inputs=+-
  Subtract_20793 : Sum  Inputs=+-
  Subtract_48823 : Sum  Inputs=+-
  Subtract_68101 : Sum  Inputs=+-
  Subtract_7f590 : Sum  Inputs=+-
  Subtract_b75d5 : Sum  Inputs=+-
  Subtract_c97a9 : Sum  Inputs=+-
  Subtract_d97f7 : Sum  Inputs=+-
  Blockout_d_w_SG_D_3_c2bca : Outport
  wires:
  Constant_x_qd_96f2d/1 -> Subtract_48823/1
  Subtract_7f590/1 -> Product_11d50/2
  Subtract_c97a9/1 -> Divide_220c7/1
  Constant_-1_d5d71/1 -> Product_400ec/1
  Add_9fc90/1 -> Product_8d6f8/2
  Constant_x_qdd_1a87d/1 -> Subtract_48823/2
  Subtract_d97f7/1 -> Product_ec500/2
  Constant_x_l_dcaac/1 -> Product_400ec/2
  State_psi_d_SG_D_3_acc7c/1 -> Add_d5b01/2
  Add_d3b90/1 -> Divide_19ae7/2
  Constant_x_dd_c3526/1 -> Subtract_b75d5/1
  Constant_x_l_f70ac/1 -> Product_e4d2d/2
  Constant_-1_f128f/1 -> Product_27356/1
  Divide_70786/1 -> Subtract_20793/2
  Constant_x_ddd_cc43f/1 -> Subtract_7f590/2
  Constant_x_qdd_c12c5/1 -> Add_9fc90/2
  Constant_pi_de4f4/1 -> Product_8c455/2
  Product_400ec/1 -> Add_9fc90/1
  Constant_-2.0_1e075/1 -> Product_4dd31/1
  Constant_-1_655c2/1 -> Product_e4d2d/1
  Constant_2.0_dc733/1 -> Product_c6131/1
  Product_4dd31/1 -> Product_66d14/1
  Constant_-1_ca6b4/1 -> Product_8a93f/1
  Subtract_07097/1 -> Add_b44f2/1
  Constant_x_l_fdf3a/1 -> Product_8a93f/2
  Constant_x_l_93dfd/1 -> Subtract_d97f7/2
  Constant_-1_aff0e/1 -> Product_d10e4/1
  State_psi_1d_SG_D_3_9d901/1 -> Product_d10e4/2
  Constant_x_dd_70460/1 -> Subtract_7f590/1
  Product_d10e4/1 -> Product_11d50/1
  State_psi_gq_SG_D_3_862a3/1 -> Product_8d6f8/1
  Constant_x_qd_f9c24/1 -> Add_d3b90/2
  Product_e4d2d/1 -> Add_d3b90/1
  State_psi_kq_SG_D_3_8659d/1 -> Product_9cc69/1
  Subtract_48823/1 -> Product_9cc69/2
  Product_c6131/1 -> Product_ef688/1
  Product_66d14/1 -> Add_fc774/1
  Product_8a93f/1 -> Add_2d3ca/1
  State_psi_q_SG_D_3_f5e8c/1 -> Product_40a83/1
  Constant_x_qd_3a749/1 -> Add_2d3ca/2
  Constant_x_l_38042/1 -> Subtract_b75d5/2
  Constant_x_ddd_025b6/1 -> Subtract_d97f7/1
  Constant_x_l_46a64/1 -> Subtract_68101/2
  Product_8d6f8/1 -> Divide_19ae7/1
  Product_9cc69/1 -> Divide_8c778/1
  Add_2d3ca/1 -> Divide_8c778/2
  Product_11d50/1 -> Divide_1eaaf/1
  Subtract_b75d5/1 -> Divide_1eaaf/2
  Constant_2.0_f0108/1 -> Product_8c455/1
  State_psi_fd_SG_D_3_07cc6/1 -> Product_ec500/1
  Constant_x_dd_415ea/1 -> Subtract_68101/1
  Divide_19ae7/1 -> Subtract_07097/1
  Product_ec500/1 -> Divide_70786/1
  Divide_8c778/1 -> Subtract_07097/2
  Divide_1eaaf/1 -> Add_d5b01/1
  Product_6dfc4/1 -> Subtract_c97a9/2
  Subtract_68101/1 -> Divide_70786/2
  Constant_pi_f332e/1 -> Product_4dd31/2
  Constant_pi_47872/1 -> Product_c6131/2
  Constant_-1_aca47/1 -> Product_89eea/1
  State_psi_d_SG_D_3_195dc/1 -> Product_89eea/2
  State_psi_q_SG_D_3_bf6de/1 -> Add_b44f2/2
  Add_d5b01/1 -> Subtract_20793/1
  Constant_f0_c9c60/1 -> Product_66d14/2
  Product_89eea/1 -> Product_536a5/1
  Add_b44f2/1 -> Product_536a5/2
  Subtract_20793/1 -> Product_40a83/2
  Constant_D_0015e/1 -> Product_27356/2
  State_w_SG_D_3_22a21/1 -> Add_fc774/2
  Product_8c455/1 -> Product_43e19/1
  State_T_m_SG_D_3_662ce/1 -> Product_43e19/2
  Product_536a5/1 -> Divide_37524/1
  Constant_x_qdd_f20dc/1 -> Divide_37524/2
  Product_40a83/1 -> Divide_3ab50/1
  Constant_x_ddd_5adab/1 -> Divide_3ab50/2
  Product_27356/1 -> Product_efaae/1
  Add_fc774/1 -> Product_efaae/2
  Product_43e19/1 -> Product_044a7/1
  Constant_f0_815f2/1 -> Product_044a7/2
  Constant_f0_adb47/1 -> Product_ef688/2
  Divide_37524/1 -> Add_75983/1
  Divide_3ab50/1 -> Add_75983/2
  Product_efaae/1 -> Add_1ddab/1
  Product_044a7/1 -> Add_1ddab/2
  Product_ef688/1 -> Product_6dfc4/1
  Add_75983/1 -> Product_6dfc4/2
  Add_1ddab/1 -> Subtract_c97a9/1
  Constant_2.0_d0be3/1 -> Product_27da9/1
  Constant_H_ccb07/1 -> Product_27da9/2
  Product_27da9/1 -> Divide_220c7/2
  Divide_220c7/1 -> Blockout_d_w_SG_D_3_c2bca/1

== system IEEE9_case/SG_D_3/i_d_SG_D_3_block ==
  note: i_d_SG_D_3 in IEEE9_case
      | $\frac{\sin\left(\theta _{\mathrm{SG},D,3}\right)\,\left(\frac{\psi _{\mathrm{1d},\mathrm{SG},D,3}\,\left(x_{\mathrm{dd}}-x_{\mathrm{ddd}}\right)}{x_{\mathrm{dd}}-x_{l}}-\psi _{d,\mathrm{SG},D,3}+\frac{\psi _{\mathrm{fd},\mathrm{SG},D,3}\,\left(x_{\mathrm{ddd}}-x_{l}\right)}{x_{\mathrm{dd}}-x_{l}}\right)}{x_{\mathrm{ddd}}}-\frac{\cos\left(\theta _{\mathrm{SG},D,3}\right)\,\left(\psi _{q,\mathrm{SG},D,3}+\frac{\psi _{\mathrm{gq},\mathrm{SG},D,3}\,\left(x_{l}-x_{\mathrm{qdd}}\right)}{x_{l}-x_{\mathrm{qd}}}+\frac{\psi _{\mathrm{kq},\mathrm{SG},D,3}\,\left(x_{\mathrm{qd}}-x_{\mathrm{qdd}}\right)}{x_{l}-x_{\mathrm{qd}}}\right)}{x_{\mathrm{qdd}}}$
      | Automatically generated on 2025-11-01 08:50:22 .
  State_psi_gq_SG_D_3_77a5e : Inport
  State_psi_kq_SG_D_3_e468d : Inport  Port=2
  State_psi_q_SG_D_3_a0a36 : Inport  Port=3
  State_theta_SG_D_3_b7be5 : Inport  Port=4
  State_psi_1d_SG_D_3_213a5 : Inport  Port=5
  State_psi_d_SG_D_3_753d5 : Inport  Port=6
  State_psi_fd_SG_D_3_e8270 : Inport  Port=7
  State_theta_SG_D_3_fbfef : Inport  Port=8
  Add_0d5d8 : Sum
  Add_5cb90 : Sum
  Add_708d9 : Sum
  Add_7419e : Sum
  Add_f2f49 : Sum
  Constant_-1_2954c : Constant  Value=-1
  Constant_-1_8148e : Constant  Value=-1
  Constant_-1_bd6ce : Constant  Value=-1
  Constant_-1_bf5dc : Constant  Value=-1
  Constant_-1_e5d70 : Constant  Value=-1
  Constant_x_dd_5257b : Constant  Value=x_dd
  Constant_x_dd_9a515 : Constant  Value=x_dd
  Constant_x_dd_aab03 : Constant  Value=x_dd
  Constant_x_ddd_95a2f : Constant  Value=x_ddd
  Constant_x_ddd_baa98 : Constant  Value=x_ddd
  Constant_x_ddd_cfb3a : Constant  Value=x_ddd
  Constant_x_l_1abaf : Constant  Value=x_l
  Constant_x_l_60c8e : Constant  Value=x_l
  Constant_x_l_71766 : Constant  Value=x_l
  Constant_x_l_942b1 : Constant  Value=x_l
  Constant_x_l_a0ecf : Constant  Value=x_l
  Constant_x_l_db185 : Constant  Value=x_l
  Constant_x_qd_4d71b : Constant  Value=x_qd
  Constant_x_qd_56164 : Constant  Value=x_qd
  Constant_x_qd_b9fd9 : Constant  Value=x_qd
  Constant_x_qdd_60a98 : Constant  Value=x_qdd
  Constant_x_qdd_c6131 : Constant  Value=x_qdd
  Constant_x_qdd_cc982 : Constant  Value=x_qdd
  Divide_3eebe : Product  Inputs=*/
  Divide_42355 : Product  Inputs=*/
  Divide_53cd3 : Product  Inputs=*/
  Divide_717ee : Product  Inputs=*/
  Divide_725b5 : Product  Inputs=*/
  Divide_ef6a2 : Product  Inputs=*/
  MathFunc_cos_2e61e : Trigonometry  Operator=cos
  MathFunc_sin_a815d : Trigonometry
  Product_01ee4 : Product
  Product_18c76 : Product
  Product_1c541 : Product
  Product_6a93c : Product
  Product_7f1f5 : Product
  Product_a0679 : Product
  Product_b2289 : Product
  Product_b56db : Product
  Product_bebc9 : Product
  Product_e944f : Product
  Product_f4a82 : Product
  Subtract_038b9 : Sum  Inputs=+-
  Subtract_1e6f4 : Sum  Inputs=+-
  Subtract_2d324 : Sum  Inputs=+-
  Subtract_45a80 : Sum  Inputs=+-
  Subtract_5f20f : Sum  Inputs=+-
  Subtract_9126c : Sum  Inputs=+-
  Subtract_a455c : Sum  Inputs=+-
  Subtract_b7ea8 : Sum  Inputs=+-
  Blockout_i_d_SG_D_3_81b50 : Outport
  wires:
  Constant_x_qd_56164/1 -> Subtract_5f20f/1
  Subtract_45a80/1 -> Blockout_i_d_SG_D_3_81b50/1
  Constant_-1_2954c/1 -> Product_b56db/1
  Constant_x_l_a0ecf/1 -> Product_01ee4/2
  Constant_x_qdd_cc982/1 -> Add_7419e/2
  Constant_x_qdd_c6131/1 -> Subtract_5f20f/2
  Constant_x_l_71766/1 -> Product_b56db/2
  Divide_53cd3/1 -> Subtract_45a80/1
  Product_b56db/1 -> Add_7419e/1
  Constant_x_ddd_baa98/1 -> Subtract_a455c/2
  Constant_-1_8148e/1 -> Product_01ee4/1
  Constant_-1_e5d70/1 -> Product_b2289/1
  Constant_x_l_1abaf/1 -> Product_b2289/2
  State_psi_1d_SG_D_3_213a5/1 -> Product_1c541/2
  State_psi_gq_SG_D_3_77a5e/1 -> Product_f4a82/1
  Product_1c541/1 -> Product_7f1f5/1
  Add_7419e/1 -> Product_f4a82/2
  Product_01ee4/1 -> Add_f2f49/1
  Constant_x_qd_b9fd9/1 -> Add_f2f49/2
  State_psi_kq_SG_D_3_e468d/1 -> Product_18c76/1
  Subtract_038b9/1 -> Divide_3eebe/2
  Subtract_5f20f/1 -> Product_18c76/2
  Product_b2289/1 -> Add_0d5d8/1
  Constant_x_ddd_95a2f/1 -> Subtract_b7ea8/1
  Constant_x_qd_4d71b/1 -> Add_0d5d8/2
  Constant_-1_bf5dc/1 -> Product_1c541/1
  Constant_x_dd_9a515/1 -> Subtract_a455c/1
  Product_f4a82/1 -> Divide_725b5/1
  Add_f2f49/1 -> Divide_725b5/2
  Product_18c76/1 -> Divide_ef6a2/1
  Add_0d5d8/1 -> Divide_ef6a2/2
  Divide_3eebe/1 -> Subtract_1e6f4/2
  Subtract_a455c/1 -> Product_7f1f5/2
  State_theta_SG_D_3_b7be5/1 -> MathFunc_cos_2e61e/1
  Constant_x_dd_5257b/1 -> Subtract_9126c/1
  Product_e944f/1 -> Product_6a93c/1
  Constant_x_l_942b1/1 -> Subtract_9126c/2
  Add_5cb90/1 -> Subtract_1e6f4/1
  Constant_x_l_60c8e/1 -> Subtract_b7ea8/2
  State_theta_SG_D_3_fbfef/1 -> MathFunc_sin_a815d/1
  Divide_725b5/1 -> Subtract_2d324/1
  Add_708d9/1 -> Product_e944f/2
  Divide_ef6a2/1 -> Subtract_2d324/2
  Product_7f1f5/1 -> Divide_42355/1
  Subtract_9126c/1 -> Divide_42355/2
  State_psi_fd_SG_D_3_e8270/1 -> Product_bebc9/1
  Divide_717ee/1 -> Subtract_45a80/2
  Subtract_b7ea8/1 -> Product_bebc9/2
  Constant_x_dd_aab03/1 -> Subtract_038b9/1
  Subtract_2d324/1 -> Add_708d9/1
  Constant_x_l_db185/1 -> Subtract_038b9/2
  Constant_-1_bd6ce/1 -> Product_e944f/1
  State_psi_q_SG_D_3_a0a36/1 -> Add_708d9/2
  Divide_42355/1 -> Add_5cb90/1
  State_psi_d_SG_D_3_753d5/1 -> Add_5cb90/2
  Product_bebc9/1 -> Divide_3eebe/1
  MathFunc_cos_2e61e/1 -> Product_6a93c/2
  MathFunc_sin_a815d/1 -> Product_a0679/2
  Subtract_1e6f4/1 -> Product_a0679/1
  Product_6a93c/1 -> Divide_53cd3/1
  Constant_x_qdd_60a98/1 -> Divide_53cd3/2
  Product_a0679/1 -> Divide_717ee/1
  Constant_x_ddd_cfb3a/1 -> Divide_717ee/2
